simulink model "one"  (R2017b)
settings: Solver=VariableStepAuto  StartTime=0.0  StopTime=30  RelTol=1e-3
values from neighbouring files (symbols this model uses):
  Cx = 52.92    [Parameters.m]
  k1_m = 5.09199    [Parameters.m]
  k2_m = 2.19    [Parameters.m]
  K_thruster = 2.89    [Parameters.m]
  lambda11 = 0.6    [Parameters.m]
  m = 24.7    [Parameters.m]
  T_thruster = 0.1    [Parameters.m]
settings Model: Creator=Eugene  LastModifiedBy=hp

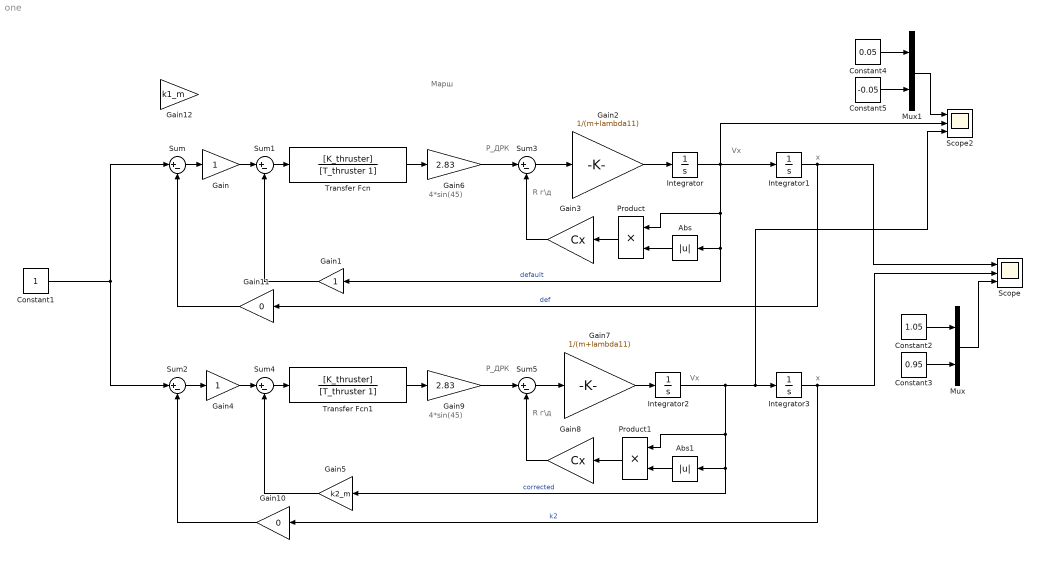
== system one ==
  note: R г\д
  note: P_ДРК
  note: 4*sin(45)
  note: Марш
  note: x
  note: Vx
  note: R г\д
  note: P_ДРК
  note: 4*sin(45)
  note: x
  note: Vx
  Abs : Abs
  Abs1 : Abs
  Constant1 : Constant
  Constant2 : Constant  Value=1.05
  Constant3 : Constant  Value=0.95
  Constant4 : Constant  Value=0.05
  Constant5 : Constant  Value=-0.05
  Gain : Gain
  Gain1 : Gain
  Gain10 : Gain  Gain=0
  Gain11 : Gain  Gain=0
  Gain12 : Gain  Gain=k1_m
  Gain2 : Gain  Gain=1/(m+lambda11)
  Gain3 : Gain  Gain=Cx
  Gain4 : Gain
  Gain5 : Gain  Gain=k2_m
  Gain6 : Gain  Gain=2.83
  Gain7 : Gain  Gain=1/(m+lambda11)
  Gain8 : Gain  Gain=Cx
  Gain9 : Gain  Gain=2.83
  Integrator{,1..3} (4 alike) : Integrator
  Mux : Mux  Inputs=2
  Mux1 : Mux  Inputs=2
  Product : Product
  Product1 : Product
  Scope : Scope  NumInputPorts=3
  Scope2 : Scope  NumInputPorts=3
  Sum{,1..5} (6 alike) : Sum  Inputs=|+-
  Transfer Fcn : TransferFcn  Numerator=[K_thruster]  Denominator=[T_thruster 1]
  Transfer Fcn1 : TransferFcn  Numerator=[K_thruster]  Denominator=[T_thruster 1]
  wires:
  Constant1/1 -> Sum2/1, Sum/1
  Sum/1 -> Gain/1
  Gain/1 -> Sum1/1
  Sum1/1 -> Transfer Fcn/1
  Gain2/1 -> Integrator/1
  Abs/1 -> Product/2
  Product/1 -> Gain3/1
  Gain3/1 -> Sum3/2
  Sum3/1 -> Gain2/1
  Transfer Fcn/1 -> Gain6/1
  Gain1/1 -> Sum1/2
  Integrator/1 -> Gain1/1, Abs/1, Product/1, Scope2/2, Integrator1/1  "default"
  Integrator1/1 -> Gain11/1, Scope/1  "def"
  Gain6/1 -> Sum3/1
  Gain9/1 -> Sum5/1
  Integrator3/1 -> Scope/2, Gain10/1  "k2"
  Integrator2/1 -> Scope2/3, Integrator3/1, Gain5/1, Abs1/1, Product1/1  "corrected"
  Gain5/1 -> Sum4/2
  Transfer Fcn1/1 -> Gain9/1
  Sum5/1 -> Gain7/1
  Gain8/1 -> Sum5/2
  Product1/1 -> Gain8/1
  Abs1/1 -> Product1/2
  Gain7/1 -> Integrator2/1
  Sum4/1 -> Transfer Fcn1/1
  Gain4/1 -> Sum4/1
  Sum2/1 -> Gain4/1
  Constant2/1 -> Mux/1
  Constant3/1 -> Mux/2
  Mux/1 -> Scope/3
  Mux1/1 -> Scope2/1
  Constant5/1 -> Mux1/2
  Constant4/1 -> Mux1/1
  Gain10/1 -> Sum2/2
  Gain11/1 -> Sum/2
